simulink model "AirCraft_Fuel_Distribution"  (R2023b)
settings: Solver=VariableStepAuto  StartTime=0.0  StopTime=8000  MaxStep=10  RelTol=1e-04  AbsTol=1e-04
undefined symbols (not defined in the file): cutoff_time_const, mover_time_constant, opening_max, pump_engine, pump_wing, rho_ref, vol_fuel_min
libraries: fl_lib x52, nesl_utility x33, SimscapeFluids_lib x17, simulink_extras x11, SignalEditorBlockLib x2
(part 2 of 2)

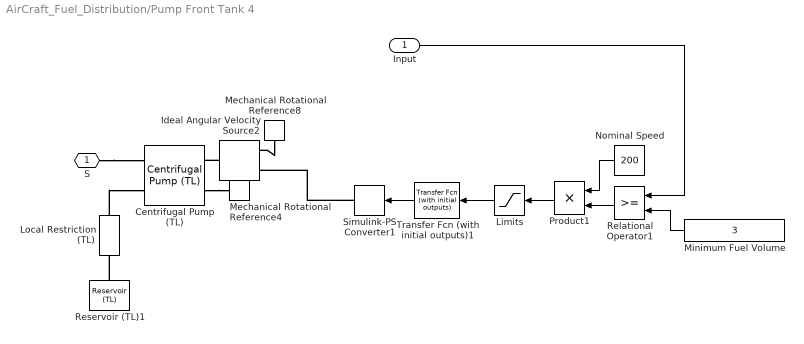
== system AirCraft_Fuel_Distribution/Pump Front Tank 4 ==
  Input : Inport
  Centrifugal Pump (TL) : SimscapeFluids_lib/Thermal Liquid/Pumps & Motors/Centrifugal Pump (TL)  pump_parameterization=1  mech_orientation=1  flow_rate_1D_TLU=pump_wing(:,1) m^3/s  head_1D_TLU=pump_wing(:,2)./(9.81*rho_ref) m  power_1D_TLU=pump_wing(:,3) W  rho_ref_1D=rho_ref kg/m^3  omega_ref_1D=omega_ref rad/s  flow_rate_2D_TLU=[16.67, 23.33, 30, 40, 53.33, 60] lpm  omega_2D_TLU=[2450, 2800, 3150, 3500] rpm  head_2D_TLU=[25, 32.7, 42.5, 50; 24, 31.7, 41, 49; 22.7, 30.5, 39, 47.5; 20, 28, 36, 45; 15.7, 24, 32, 40; 12.5, 21, 29.5, 37.5] m  power_2D_TLU=[.28, .38, .5, .6; .31, .41, .55, .68; .33, .44, .6, .75; .36, .48, .65, .83; .38, .53, .72, .93; .39, .55, .75, .97] kW  rho_ref_2D=920 kg/m^3  omega_threshold=omega_threshold rad/s  area=area_pipe m^2  mdot_A_specify=off  mdot_A_priority=None  mdot_A=1 kg/s  mdot_A_nominal_specify=off  mdot_A_nominal_unit=kg/s  mdot_A_nominal_value=1
      settings: InternalSimscapePortConfiguration="{\"Bottom\":[],\"Left\":[{\"id\":\"A\",\"label\":\"A\",\"type\":\"foundation.thermal_liquid.thermal_liquid\"},{\"id\":\"B\",\"label\":\"B\",\"type\":\"foundation.thermal_liquid.thermal_liquid\"}],\"Right\":[{\"id\":\"R\",\"label\":\"R\",\"type\":\"foundation.mechanical.rotational.rotational\"},{\"id\":\"C\",\"label\":\"C\",\"type\":\"foundation.mechanical.rotational.rotational\"}],\"Top\":[]}"
  Ideal Angular Velocity Source2 : fl_lib/Mechanical/Mechanical Sources/Ideal Angular Velocity Source
  Limits : Saturate  UpperLimit=200  LowerLimit=20
  Local Restriction (TL) : fl_lib/Thermal Liquid/Elements/Local Restriction (TL)  restriction_type=foundation.enum.restriction_type.fixed  restriction_area=1e-4 m^2  min_area=1e-10 m^2  max_area=0.005 m^2  area=1e-3 m^2  Cd=0.7  pressure_recovery=simscape.enum.onoff.on  Re_c=12
  Mechanical Rotational Reference4 : fl_lib/Mechanical/Rotational Elements/Mechanical Rotational Reference
  Mechanical Rotational Reference8 : fl_lib/Mechanical/Rotational Elements/Mechanical Rotational Reference
  Minimum Fuel Volume : Constant  Value=3
  Nominal Speed : Constant  Value=200
  Product1 : Product  RndMeth=Zero
  Relational Operator1 : RelationalOperator  OutDataTypeStr=boolean  InputSameDT=off
  Reservoir (TL)1 : fl_lib/Thermal Liquid/Elements/Reservoir (TL)  pressure_spec=2  reservoir_pressure=0.1 MPa  reservoir_temperature=273.15+60 K  area=0.01 m^2
  Simulink-PS Converter1 : nesl_utility/Simulink-PS Converter  PhysicalDomain=network_engine_domain  SubClassName=ps_input  LeftPortType=input  RightPortType=output  PseudoPeriodic=off  Frequencies=[]  NoiseDistribution=none  NoiseParameters=[]  Unit=rev/s  AffineConversion=off  FilteringAndDerivatives=provide  SimscapeFilterOrder=1  InputFilterTimeConstant=0.001  UdotUserProvided=0
  Transfer Fcn (with initial outputs)1 : simulink_extras/Additional Linear/Transfer Fcn (with initial outputs)  N=[1]  D=[2 1]  Y0=0  U0=0
  S : PMIOPort  Side=Left
  wires:
  Nominal Speed/1 -> Product1/1
  Relational Operator1/1 -> Product1/2
  Transfer Fcn (with initial outputs)1/1 -> Simulink-PS Converter1/1
  Product1/1 -> Limits/1
  Minimum Fuel Volume/1 -> Relational Operator1/2
  Limits/1 -> Transfer Fcn (with initial outputs)1/1
  Input/1 -> Relational Operator1/1
  connections:
  Centrifugal Pump (TL)/RConn2 -- Mechanical Rotational Reference4/LConn1
  Reservoir (TL)1/LConn1 -- Local Restriction (TL)/RConn1
  Ideal Angular Velocity Source2/LConn1 -- Centrifugal Pump (TL)/RConn1
  Mechanical Rotational Reference8/LConn1 -- Ideal Angular Velocity Source2/RConn2
  Simulink-PS Converter1/RConn1 -- Ideal Angular Velocity Source2/RConn1
  S/RConn1 -- Centrifugal Pump (TL)/LConn1
  Local Restriction (TL)/LConn1 -- Centrifugal Pump (TL)/LConn2

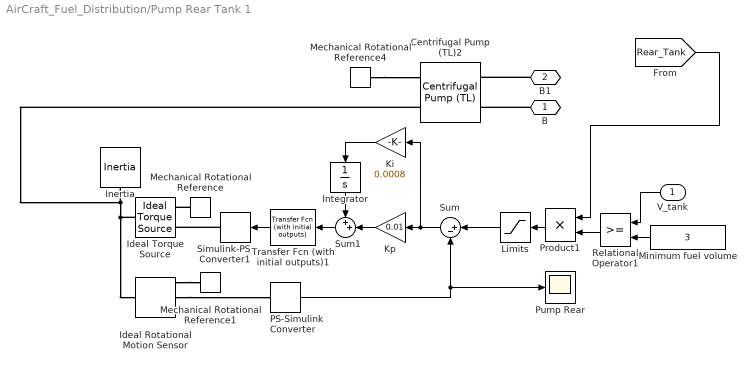
== system AirCraft_Fuel_Distribution/Pump Rear Tank 1 ==
  V_tank : Inport
  Centrifugal Pump (TL)2 : SimscapeFluids_lib/Thermal Liquid/Pumps & Motors/Centrifugal Pump (TL)  pump_parameterization=1  mech_orientation=1  flow_rate_1D_TLU=pump_wing(:,1) m^3/s  head_1D_TLU=pump_wing(:,2)./(9.81*rho_ref) m  power_1D_TLU=pump_wing(:,3) W  rho_ref_1D=rho_ref kg/m^3  omega_ref_1D=omega_ref rad/s  flow_rate_2D_TLU=[16.67, 23.33, 30, 40, 53.33, 60] lpm  omega_2D_TLU=[2450, 2800, 3150, 3500] rpm  head_2D_TLU=[25, 32.7, 42.5, 50; 24, 31.7, 41, 49; 22.7, 30.5, 39, 47.5; 20, 28, 36, 45; 15.7, 24, 32, 40; 12.5, 21, 29.5, 37.5] m  power_2D_TLU=[.28, .38, .5, .6; .31, .41, .55, .68; .33, .44, .6, .75; .36, .48, .65, .83; .38, .53, .72, .93; .39, .55, .75, .97] kW  rho_ref_2D=920 kg/m^3  omega_threshold=omega_threshold rad/s  area=area_pipe m^2  mdot_A_specify=off  mdot_A_priority=None  mdot_A=1 kg/s  mdot_A_nominal_specify=off  mdot_A_nominal_unit=kg/s  mdot_A_nominal_value=1
      settings: InternalSimscapePortConfiguration="{\"Bottom\":[],\"Left\":[{\"id\":\"A\",\"label\":\"A\",\"type\":\"foundation.thermal_liquid.thermal_liquid\"},{\"id\":\"B\",\"label\":\"B\",\"type\":\"foundation.thermal_liquid.thermal_liquid\"}],\"Right\":[{\"id\":\"R\",\"label\":\"R\",\"type\":\"foundation.mechanical.rotational.rotational\"},{\"id\":\"C\",\"label\":\"C\",\"type\":\"foundation.mechanical.rotational.rotational\"}],\"Top\":[]}"
  Ideal Rotational Motion Sensor : fl_lib/Mechanical/Mechanical Sensors/Ideal Rotational Motion Sensor  wrap_angle=simscape.enum.onoff.off  offset=0 rad
  Ideal Torque Source : fl_lib/Mechanical/Mechanical Sources/Ideal Torque Source
  Inertia : fl_lib/Mechanical/Rotational Elements/Inertia  inertia=0.005 kg*m^2  w_specify=on  w_priority=High  w=omega_min rev/s  w_nominal_specify=off  w_nominal_unit=rad/s  w_nominal_value=1  t_specify=off  t_priority=None  t=0 N*m  t_nominal_specify=off  t_nominal_unit=N*m  t_nominal_value=1
  Integrator : Integrator  LimitOutput=on  UpperSaturationLimit=1  LowerSaturationLimit=-1
  Ki : Gain  Gain=0.0008
  Kp : Gain  Gain=0.01
  Limits : Saturate  UpperLimit=250  LowerLimit=20
  Mechanical Rotational Reference : fl_lib/Mechanical/Rotational Elements/Mechanical Rotational Reference
  Mechanical Rotational Reference1 : fl_lib/Mechanical/Rotational Elements/Mechanical Rotational Reference
  Mechanical Rotational Reference4 : fl_lib/Mechanical/Rotational Elements/Mechanical Rotational Reference
  Minimum fuel volume : Constant  Value=3
  PS-Simulink Converter : nesl_utility/PS-Simulink Converter  PhysicalDomain=network_engine_domain  SubClassName=ps_output  LeftPortType=input  RightPortType=output  PseudoPeriodic=off  Frequencies=[]  Unit=rev/s  AffineConversion=off
  Product1 : Product  RndMeth=Zero
  Pump Rear : Scope
  Relational Operator1 : RelationalOperator  OutDataTypeStr=boolean  InputSameDT=off
  Simulink-PS Converter1 : nesl_utility/Simulink-PS Converter  PhysicalDomain=network_engine_domain  SubClassName=ps_input  LeftPortType=input  RightPortType=output  PseudoPeriodic=off  Frequencies=[]  NoiseDistribution=none  NoiseParameters=[]  Unit=N*m  AffineConversion=off  FilteringAndDerivatives=provide  SimscapeFilterOrder=1  InputFilterTimeConstant=0.001  UdotUserProvided=0
  Sum : Sum  Inputs=|+-
  Sum1 : Sum  Inputs=++|
  Transfer Fcn (with initial outputs)1 : simulink_extras/Additional Linear/Transfer Fcn (with initial outputs)  N=[1]  D=[mover_time_constant 1]  Y0=0  U0=0
  B : PMIOPort  Side=Left
  B1 : PMIOPort  Port=2  Side=Left
  wires:
  Product1/1 -> Limits/1
  Ki/1 -> Integrator/1
  Integrator/1 -> Sum1/1
  Kp/1 -> Sum1/2
  Transfer Fcn (with initial outputs)1/1 -> Simulink-PS Converter1/1
  Limits/1 -> Sum/1
  Sum1/1 -> Transfer Fcn (with initial outputs)1/1
  Minimum fuel volume/1 -> Relational Operator1/2
  Sum/1 -> Ki/1, Kp/1
  PS-Simulink Converter/1 -> Pump Rear/1, Sum/2
  V_tank/1 -> Relational Operator1/1
  Relational Operator1/1 -> Product1/2
  [Rear_Tank] -> Product1/1
  connections:
  Mechanical Rotational Reference4/LConn1 -- Centrifugal Pump (TL)2/RConn2
  B1/RConn1 -- Centrifugal Pump (TL)2/LConn2
  B/RConn1 -- Centrifugal Pump (TL)2/LConn1
  Inertia/LConn1 -- Ideal Rotational Motion Sensor/LConn1 -- Ideal Torque Source/LConn1 -- Centrifugal Pump (TL)2/RConn1
  Ideal Rotational Motion Sensor/RConn1 -- Mechanical Rotational Reference1/LConn1
  Mechanical Rotational Reference/LConn1 -- Ideal Torque Source/RConn2
  Simulink-PS Converter1/RConn1 -- Ideal Torque Source/RConn1
  Ideal Rotational Motion Sensor/RConn2 -- PS-Simulink Converter/LConn1

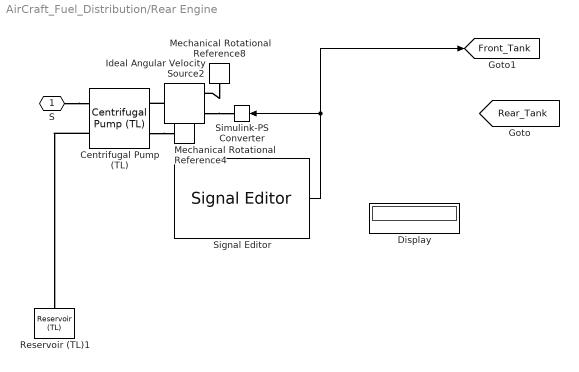
== system AirCraft_Fuel_Distribution/Rear Engine ==
  Centrifugal Pump (TL) : SimscapeFluids_lib/Thermal Liquid/Pumps & Motors/Centrifugal Pump (TL)  pump_parameterization=1  mech_orientation=1  flow_rate_1D_TLU=pump_engine(:,1) m^3/s  head_1D_TLU=pump_engine(:,2)./(9.81*rho_ref) m  power_1D_TLU=pump_engine(:,3) W  rho_ref_1D=rho_ref kg/m^3  omega_ref_1D=omega_ref rad/s  flow_rate_2D_TLU=[16.67, 23.33, 30, 40, 53.33, 60] lpm  omega_2D_TLU=[2450, 2800, 3150, 3500] rpm  head_2D_TLU=[25, 32.7, 42.5, 50; 24, 31.7, 41, 49; 22.7, 30.5, 39, 47.5; 20, 28, 36, 45; 15.7, 24, 32, 40; 12.5, 21, 29.5, 37.5] m  power_2D_TLU=[.28, .38, .5, .6; .31, .41, .55, .68; .33, .44, .6, .75; .36, .48, .65, .83; .38, .53, .72, .93; .39, .55, .75, .97] kW  rho_ref_2D=920 kg/m^3  omega_threshold=omega_threshold rad/s  area=area_pipe m^2  mdot_A_specify=off  mdot_A_priority=None  mdot_A=1 kg/s  mdot_A_nominal_specify=off  mdot_A_nominal_unit=kg/s  mdot_A_nominal_value=1
      settings: InternalSimscapePortConfiguration="{\"Bottom\":[],\"Left\":[{\"id\":\"A\",\"label\":\"A\",\"type\":\"foundation.thermal_liquid.thermal_liquid\"},{\"id\":\"B\",\"label\":\"B\",\"type\":\"foundation.thermal_liquid.thermal_liquid\"}],\"Right\":[{\"id\":\"R\",\"label\":\"R\",\"type\":\"foundation.mechanical.rotational.rotational\"},{\"id\":\"C\",\"label\":\"C\",\"type\":\"foundation.mechanical.rotational.rotational\"}],\"Top\":[]}"
  Display : Display
  Ideal Angular Velocity Source2 : fl_lib/Mechanical/Mechanical Sources/Ideal Angular Velocity Source
  Mechanical Rotational Reference4 : fl_lib/Mechanical/Rotational Elements/Mechanical Rotational Reference
  Mechanical Rotational Reference8 : fl_lib/Mechanical/Rotational Elements/Mechanical Rotational Reference
  Reservoir (TL)1 : fl_lib/Thermal Liquid/Elements/Reservoir (TL)  pressure_spec=2  reservoir_pressure=0.1 MPa  reservoir_temperature=273.15+60 K  area=0.01 m^2
  Signal Editor : SignalEditorBlockLib/Signal Editor  FileName=Scenario1_Consumption.mat  ActiveScenario=Scenario1  ActiveSignal=Rear Tank  IsBus=off  OutputBusObjectStr=Bus: BusObject  SampleTime=0  Interpolate=off  ZeroCross=off  OutputAfterFinalValue=Setting to zero  Unit=inherit  PreserveSignalName=on  ApplySigPropsToAllScenarios=on  ApplySigPropsToAllSignals=off
  Simulink-PS Converter : nesl_utility/Simulink-PS Converter  PhysicalDomain=network_engine_domain  SubClassName=ps_input  LeftPortType=input  RightPortType=output  PseudoPeriodic=off  Frequencies=[]  NoiseDistribution=none  NoiseParameters=[]  Unit=1  AffineConversion=off  FilteringAndDerivatives=provide  SimscapeFilterOrder=1  InputFilterTimeConstant=0.001  UdotUserProvided=0
  S : PMIOPort  Side=Right
  tag scope: Front_Tank=global, Rear_Tank=global
  wires:
  Signal Editor/1 -> [Front_Tank], Simulink-PS Converter/1
  ? -> Display/1, [Rear_Tank]
  connections:
  Centrifugal Pump (TL)/LConn2 -- Reservoir (TL)1/LConn1
  Mechanical Rotational Reference8/LConn1 -- Ideal Angular Velocity Source2/RConn2
  Ideal Angular Velocity Source2/LConn1 -- Centrifugal Pump (TL)/RConn1
  Centrifugal Pump (TL)/RConn2 -- Mechanical Rotational Reference4/LConn1
  S/RConn1 -- Centrifugal Pump (TL)/LConn1
  Ideal Angular Velocity Source2/RConn1 -- Simulink-PS Converter/RConn1

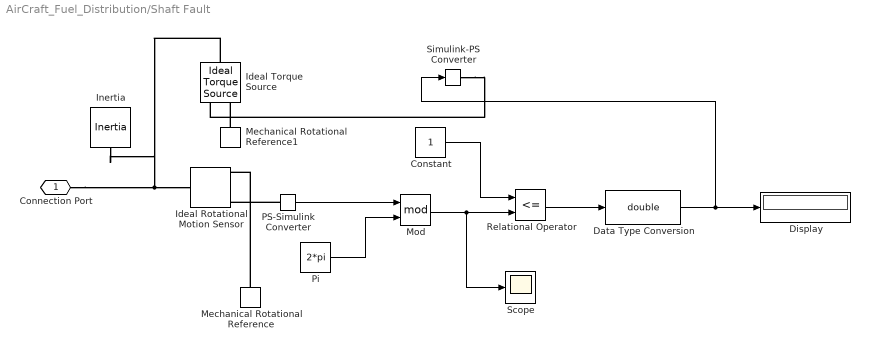
== system AirCraft_Fuel_Distribution/Shaft Fault  ==
  Constant : Constant
  Data Type Conversion : DataTypeConversion  OutDataTypeStr=double  SaturateOnIntegerOverflow=off  RndMeth=Floor
  Display : Display
  Ideal Rotational Motion Sensor : fl_lib/Mechanical/Mechanical Sensors/Ideal Rotational Motion Sensor  wrap_angle=simscape.enum.onoff.off  offset=0 rad
  Ideal Torque Source : fl_lib/Mechanical/Mechanical Sources/Ideal Torque Source
  Inertia : fl_lib/Mechanical/Rotational Elements/Inertia  inertia=0.005 kg*m^2  w_specify=on  w_priority=High  w=omega_min rev/s  w_nominal_specify=off  w_nominal_unit=rad/s  w_nominal_value=1  t_specify=off  t_priority=None  t=0 N*m  t_nominal_specify=off  t_nominal_unit=N*m  t_nominal_value=1
  Mechanical Rotational Reference : fl_lib/Mechanical/Rotational Elements/Mechanical Rotational Reference
  Mechanical Rotational Reference1 : fl_lib/Mechanical/Rotational Elements/Mechanical Rotational Reference
  Mod : Math  Operator=mod
  PS-Simulink Converter : nesl_utility/PS-Simulink Converter  PhysicalDomain=network_engine_domain  SubClassName=ps_output  LeftPortType=input  RightPortType=output  PseudoPeriodic=off  Frequencies=[]  Unit=inherit  AffineConversion=off
  Pi : Constant  Value=2*pi  OutDataTypeStr=Inherit: Inherit via back propagation
  Relational Operator : RelationalOperator  Operator=<=  OutDataTypeStr=boolean  RndMeth=Simplest  InputSameDT=off
  Scope : Scope
  Simulink-PS Converter : nesl_utility/Simulink-PS Converter  PhysicalDomain=network_engine_domain  SubClassName=ps_input  LeftPortType=input  RightPortType=output  PseudoPeriodic=off  Frequencies=[]  NoiseDistribution=none  NoiseParameters=[]  Unit=1  AffineConversion=off  FilteringAndDerivatives=provide  SimscapeFilterOrder=1  InputFilterTimeConstant=0.001  UdotUserProvided=0
  Connection Port : PMIOPort  Side=Left
  wires:
  PS-Simulink Converter/1 -> Mod/1
  Pi/1 -> Mod/2
  Mod/1 -> Scope/1, Relational Operator/2
  Constant/1 -> Relational Operator/1
  Relational Operator/1 -> Data Type Conversion/1
  Data Type Conversion/1 -> Simulink-PS Converter/1, Display/1
  connections:
  PS-Simulink Converter/LConn1 -- Ideal Rotational Motion Sensor/RConn3
  Mechanical Rotational Reference/LConn1 -- Ideal Rotational Motion Sensor/RConn1
  Connection Port/RConn1 -- Inertia/LConn1 -- Ideal Torque Source/LConn1 -- Ideal Rotational Motion Sensor/LConn1
  Simulink-PS Converter/RConn1 -- Ideal Torque Source/RConn1
  Mechanical Rotational Reference1/LConn1 -- Ideal Torque Source/RConn2

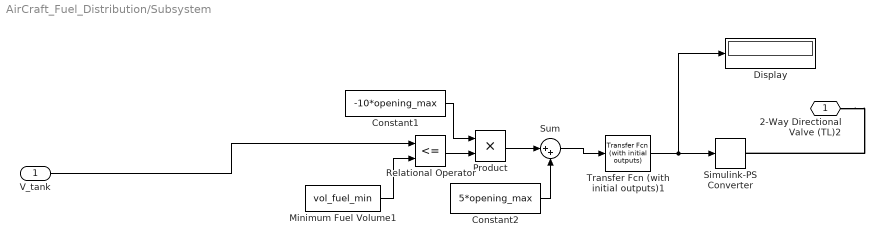
== system AirCraft_Fuel_Distribution/Subsystem ==
  V_tank : Inport
  Constant1 : Constant  Value=-10*opening_max
  Constant2 : Constant  Value=5*opening_max
  Display : Display
  Minimum Fuel Volume1 : Constant  Value=vol_fuel_min
  Product : Product  RndMeth=Zero
  Relational Operator : RelationalOperator  Operator=<=  OutDataTypeStr=boolean  InputSameDT=off
  Simulink-PS Converter : nesl_utility/Simulink-PS Converter  PhysicalDomain=network_engine_domain  SubClassName=ps_input  LeftPortType=input  RightPortType=output  PseudoPeriodic=off  Frequencies=[]  NoiseDistribution=none  NoiseParameters=[]  Unit=m  AffineConversion=off  FilteringAndDerivatives=provide  SimscapeFilterOrder=1  InputFilterTimeConstant=0.001  UdotUserProvided=0
  Sum : Sum  Inputs=|++
  Transfer Fcn (with initial outputs)1 : simulink_extras/Additional Linear/Transfer Fcn (with initial outputs)  N=[1]  D=[cutoff_time_const 1]  Y0=0  U0=0
  2-Way Directional Valve (TL)2 : PMIOPort  Side=Left
  wires:
  Constant2/1 -> Sum/2
  V_tank/1 -> Relational Operator/1
  Relational Operator/1 -> Product/2
  Product/1 -> Sum/1
  Constant1/1 -> Product/1
  Minimum Fuel Volume1/1 -> Relational Operator/2
  Sum/1 -> Transfer Fcn (with initial outputs)1/1
  Transfer Fcn (with initial outputs)1/1 -> Display/1, Simulink-PS Converter/1
  connections:
  2-Way Directional Valve (TL)2/RConn1 -- Simulink-PS Converter/RConn1

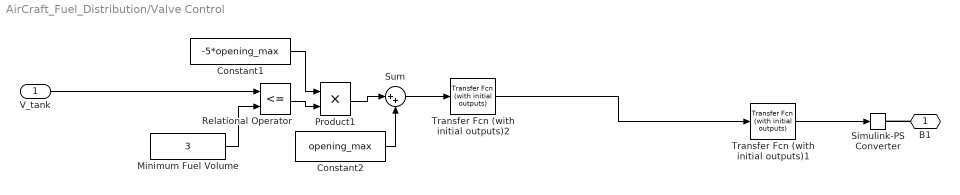
== system AirCraft_Fuel_Distribution/Valve Control ==
  V_tank : Inport
  Constant1 : Constant  Value=-5*opening_max
  Constant2 : Constant  Value=opening_max
  Minimum Fuel Volume : Constant  Value=3
  Product1 : Product  RndMeth=Zero
  Relational Operator : RelationalOperator  Operator=<=  OutDataTypeStr=boolean  ZeroCross=off  InputSameDT=off
  Simulink-PS Converter : nesl_utility/Simulink-PS Converter  PhysicalDomain=network_engine_domain  SubClassName=ps_input  LeftPortType=input  RightPortType=output  PseudoPeriodic=off  Frequencies=[]  NoiseDistribution=none  NoiseParameters=[]  Unit=1  AffineConversion=off  FilteringAndDerivatives=provide  SimscapeFilterOrder=1  InputFilterTimeConstant=0.001  UdotUserProvided=0
  Sum : Sum  Inputs=|++
  Transfer Fcn (with initial outputs)1 : simulink_extras/Additional Linear/Transfer Fcn (with initial outputs)  N=[1]  D=[cutoff_time_const 1]  Y0=0  U0=0
  Transfer Fcn (with initial outputs)2 : simulink_extras/Additional Linear/Transfer Fcn (with initial outputs)  N=[1]  D=[cutoff_time_const 1]  Y0=0  U0=0
  B1 : PMIOPort  Side=Right
  wires:
  Transfer Fcn (with initial outputs)1/1 -> Simulink-PS Converter/1
  Constant1/1 -> Product1/1
  V_tank/1 -> Relational Operator/1
  Minimum Fuel Volume/1 -> Relational Operator/2
  Constant2/1 -> Sum/2
  Product1/1 -> Sum/1
  Sum/1 -> Transfer Fcn (with initial outputs)2/1
  Relational Operator/1 -> Product1/2
  Transfer Fcn (with initial outputs)2/1 -> Transfer Fcn (with initial outputs)1/1
  connections:
  B1/RConn1 -- Simulink-PS Converter/RConn1

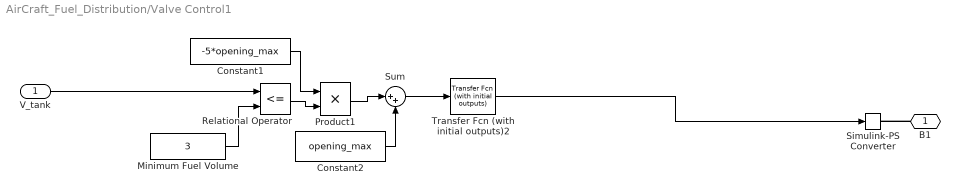
== system AirCraft_Fuel_Distribution/Valve Control1 ==
  V_tank : Inport
  Constant1 : Constant  Value=-5*opening_max
  Constant2 : Constant  Value=opening_max
  Minimum Fuel Volume : Constant  Value=3
  Product1 : Product  RndMeth=Zero
  Relational Operator : RelationalOperator  Operator=<=  OutDataTypeStr=boolean  InputSameDT=off
  Simulink-PS Converter : nesl_utility/Simulink-PS Converter  PhysicalDomain=network_engine_domain  SubClassName=ps_input  LeftPortType=input  RightPortType=output  PseudoPeriodic=off  Frequencies=[]  NoiseDistribution=none  NoiseParameters=[]  Unit=1  AffineConversion=off  FilteringAndDerivatives=provide  SimscapeFilterOrder=1  InputFilterTimeConstant=0.001  UdotUserProvided=0
  Sum : Sum  Inputs=|++
  Transfer Fcn (with initial outputs)2 : simulink_extras/Additional Linear/Transfer Fcn (with initial outputs)  N=[1]  D=[cutoff_time_const 1]  Y0=0  U0=0
  B1 : PMIOPort  Side=Left
  wires:
  V_tank/1 -> Relational Operator/1
  Constant2/1 -> Sum/2
  Minimum Fuel Volume/1 -> Relational Operator/2
  Product1/1 -> Sum/1
  Sum/1 -> Transfer Fcn (with initial outputs)2/1
  Constant1/1 -> Product1/1
  Relational Operator/1 -> Product1/2
  Transfer Fcn (with initial outputs)2/1 -> Simulink-PS Converter/1
  connections:
  B1/RConn1 -- Simulink-PS Converter/RConn1

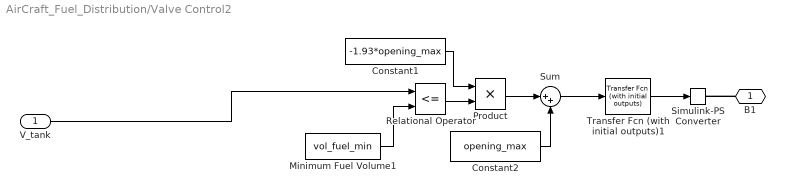
== system AirCraft_Fuel_Distribution/Valve Control2 ==
  V_tank : Inport
  Constant1 : Constant  Value=-1.93*opening_max
  Constant2 : Constant  Value=opening_max
  Minimum Fuel Volume1 : Constant  Value=vol_fuel_min
  Product : Product  RndMeth=Zero
  Relational Operator : RelationalOperator  Operator=<=  OutDataTypeStr=boolean  InputSameDT=off
  Simulink-PS Converter : nesl_utility/Simulink-PS Converter  PhysicalDomain=network_engine_domain  SubClassName=ps_input  LeftPortType=input  RightPortType=output  PseudoPeriodic=off  Frequencies=[]  NoiseDistribution=none  NoiseParameters=[]  Unit=1  AffineConversion=off  FilteringAndDerivatives=provide  SimscapeFilterOrder=1  InputFilterTimeConstant=0.001  UdotUserProvided=0
  Sum : Sum  Inputs=|++
  Transfer Fcn (with initial outputs)1 : simulink_extras/Additional Linear/Transfer Fcn (with initial outputs)  N=[1]  D=[cutoff_time_const 1]  Y0=0  U0=0
  B1 : PMIOPort  Side=Right
  wires:
  Sum/1 -> Transfer Fcn (with initial outputs)1/1
  Product/1 -> Sum/1
  Constant2/1 -> Sum/2
  Minimum Fuel Volume1/1 -> Relational Operator/2
  Constant1/1 -> Product/1
  V_tank/1 -> Relational Operator/1
  Relational Operator/1 -> Product/2
  Transfer Fcn (with initial outputs)1/1 -> Simulink-PS Converter/1
  connections:
  B1/RConn1 -- Simulink-PS Converter/RConn1

== system AirCraft_Fuel_Distribution/Valve Control3 ==
  V_tank : Inport
  Constant : Constant  Value=-1.93*opening_max
  Constant2 : Constant  Value=opening_max
  Minimum Fuel Volume : Constant  Value=vol_fuel_min
  Product : Product  RndMeth=Zero
  Relational Operator : RelationalOperator  Operator=<=  OutDataTypeStr=boolean  InputSameDT=off
  Simulink-PS Converter : nesl_utility/Simulink-PS Converter  PhysicalDomain=network_engine_domain  SubClassName=ps_input  LeftPortType=input  RightPortType=output  PseudoPeriodic=off  Frequencies=[]  NoiseDistribution=none  NoiseParameters=[]  Unit=1  AffineConversion=off  FilteringAndDerivatives=provide  SimscapeFilterOrder=1  InputFilterTimeConstant=0.001  UdotUserProvided=0
  Sum : Sum  Inputs=|++
  Transfer Fcn (with initial outputs)1 : simulink_extras/Additional Linear/Transfer Fcn (with initial outputs)  N=[1]  D=[cutoff_time_const 1]  Y0=0  U0=0
  B1 : PMIOPort  Side=Left
  wires:
  Constant/1 -> Product/1
  Transfer Fcn (with initial outputs)1/1 -> Simulink-PS Converter/1
  V_tank/1 -> Relational Operator/1
  Relational Operator/1 -> Product/2
  Minimum Fuel Volume/1 -> Relational Operator/2
  Constant2/1 -> Sum/2
  Product/1 -> Sum/1
  Sum/1 -> Transfer Fcn (with initial outputs)1/1
  connections:
  B1/RConn1 -- Simulink-PS Converter/RConn1
